simulink model "lab4_1"  (R2013a)
settings: Solver=ode45  StartTime=0.0  StopTime=10.0  RelTol=1e-3
settings Model: Creator=u_labelectro  LastModifiedBy=u_labelectro

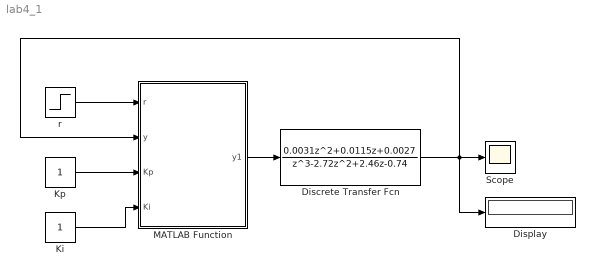
== system lab4_1 ==
  Discrete Transfer Fcn : DiscreteTransferFcn  Numerator=[0.0031 0.0115 0.0027]  Denominator=[1 -2.72 2.46 -0.74]  SampleTime=0.01
  Display : Display
  Ki : Constant
  Kp : Constant
  MATLAB Function : MATLAB Function  TreatAsAtomicUnit=on
  Scope : Scope
  r : Step  SampleTime=0
  wires:
  Kp/1 -> MATLAB Function/3(Kp)
  Ki/1 -> MATLAB Function/4(Ki)
  r/1 -> MATLAB Function/1(r)
  MATLAB Function/1(y1) -> Discrete Transfer Fcn/1
  Discrete Transfer Fcn/1 -> Display/1, MATLAB Function/2(y), Scope/1

== matlab function lab4_1/MATLAB Function ==
  data: r input; y input; Kp input; Ki input; y1 output
function y1 = controlador_PI(r,y,Kp,Ki)

T = 0.01;

persistent e_ant;
persistent u_ant;

if isempty(u_ant)
    u_ant = 0;
    e_ant = 0;
end

e_act = r - y;
Akp = (e_act - e_ant)*Kp;
Aki = e_act*Ki*T;

u_act = u_ant + Akp + Aki;

e_ant = e_act;
u_ant = u_act;

end
